simulink library "libbha_parts_bellows"  (R2013b)
settings: Solver=FixedStepDiscrete  StartTime=0.0  StopTime=Inf  FixedStep=0.004  RelTol=1e-3
PostLoadFcn:
  | , if any(exist('dsrtsu_mdlpostloadfcn', 'file') == [2, 3, 6]), try dsrtsu_mdlpostloadfcn('Execute', bdroot); catch fprintf('Error in PostLoadFcn (dsrtsu_mdlpostloadfcn) for model "%s":\n %s\n', bdroot, lasterr); end, end,
undefined symbols (not defined in the file or in its folder): DiscIntNeverNeededParam, p1i
libraries: libbha_parts_bellows x4, libbha_parameters x1
settings Model: DSRTSU_INTERNAL_RTI_VER=440  DSRTSU_INTERNAL_RTI_TYPE=rti1005  DSRTSU_INTERNAL_RTIFPGA=30  Creator=Falkenhahn  LastModifiedBy=fav

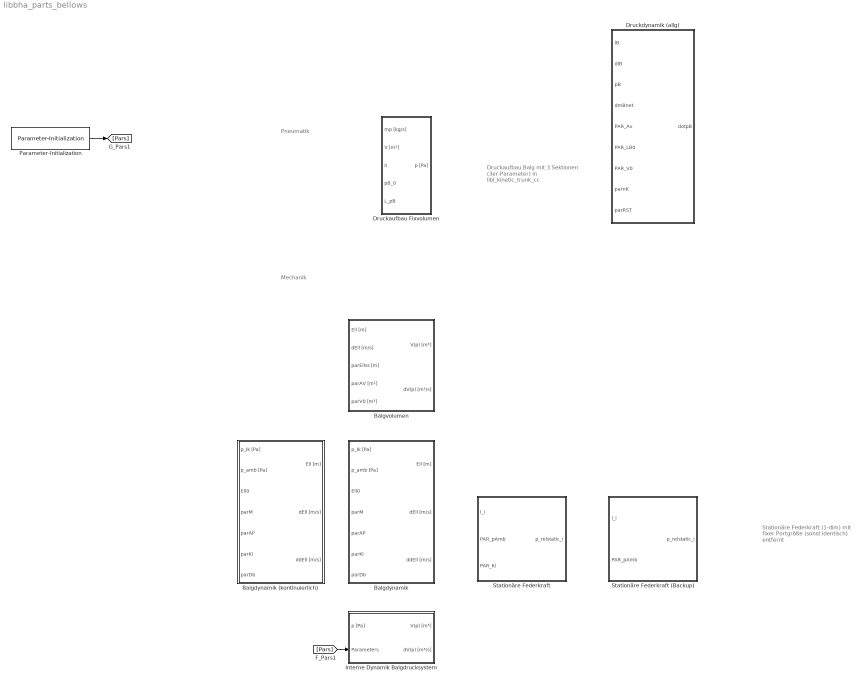
== system libbha_parts_bellows ==
  note: Stationäre Federkraft (1-dim)
      | mit fixer Portgröße (sonst identisch)
      | entfernt
  note: Druckaufbau Balg mit 3 Sektionen
      | (3er-Parameter) in
      | libl_kinetic_trunk_cc
  note: Mechanik
  note: Pneumatik
  Balgdynamik : Subsystem
  Balgdynamik (kontinuierlich) : Subsystem
      settings: AttributesFormatString=|
      | kontinuierliche Integratoren
      | (nicht geeignet für RTW)
  Balgvolumen : Subsystem
  Druckaufbau Fixvolumen : Subsystem  mask{R=288, T0=293.15}
  Druckdynamik (allg) : MATLAB Function  TreatAsAtomicUnit=on
  Interne Dynamik Balgdrucksystem : Subsystem
  Parameter-Initialization : libbha_parameters/Parameter-Initialization  bha_var_choice=BHA  tA=CONST.tA
      settings: AttributesFormatString=|
      | BHA-Variable: %<bha_var_choice>
      | sample time: %<tA>
  Stationäre Federkraft : Subsystem
      settings: AttributesFormatString=|
      | Federkennlinie als Interpolation mittels
      | Polynom 3. Ordnung mit balgspezifischen
      | Parametern p0 (konst) bis p3 (kubisch)
  Stationäre Federkraft (Backup) : Subsystem
      settings: AttributesFormatString=Federkennlinie fest einprogrammiert
  wires:
  Parameter-Initialization/1 -> [Pars]
  [Pars] -> Interne Dynamik Balgdrucksystem/2(Parameters)

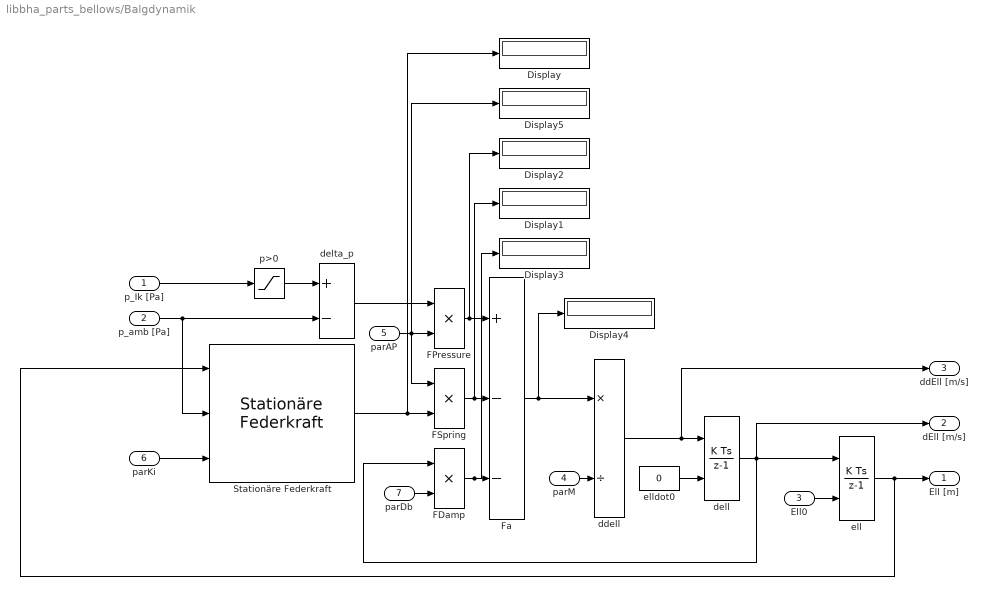
== system libbha_parts_bellows/Balgdynamik ==
  p_Ik [Pa] : Inport
  p_amb [Pa] : Inport  Port=2
  Ell0 : Inport  Port=3
  parM : Inport  Port=4
  parAP : Inport  Port=5
  parKi : Inport  Port=6
      settings: AttributesFormatString=|
      | n x 4
      | n = dim(l)
  parDb : Inport  Port=7
  Display{,1..5} (6 alike) : Display
  FDamp : Product  Inputs=**  OutDataTypeStr=Inherit: Same as first input
  FPressure : Product  Inputs=**  OutDataTypeStr=Inherit: Same as first input
  FSpring : Product  Inputs=**  OutDataTypeStr=Inherit: Same as first input
  Fa : Sum  Inputs=+--  OutDataTypeStr=Inherit: Same as first input
  Stationäre Federkraft : libbha_parts_bellows/Stationäre Federkraft
  ddell : Product  Inputs=*/  OutDataTypeStr=Inherit: Same as first input
  dell : DiscreteIntegrator  InitialConditionSource=external  SampleTime=-1  ICPrevOutput=DiscIntNeverNeededParam  ICPrevScaledInput=DiscIntNeverNeededParam
  delta_p : Sum  Inputs=+-  OutDataTypeStr=Inherit: Same as first input
  ell : DiscreteIntegrator  InitialConditionSource=external  SampleTime=-1  ICPrevOutput=DiscIntNeverNeededParam  ICPrevScaledInput=DiscIntNeverNeededParam
  elldot0 : Constant  Value=0
  p>0 : Saturate  UpperLimit=inf  LowerLimit=0.001e5
  Ell [m] : Outport
  dEll [m/s] : Outport  Port=2
  ddEll [m/s] : Outport  Port=3
  wires:
  Stationäre Federkraft/1 -> Display/1, FSpring/2
  parAP/1 -> FPressure/2, Display5/1, FSpring/1
  parDb/1 -> FDamp/2
  ddell/1 -> dell/1, ddEll [m/s]/1
  parM/1 -> ddell/2
  Fa/1 -> Display4/1, ddell/1
  FPressure/1 -> Display2/1, Fa/1
  p_Ik [Pa]/1 -> p>0/1
  p_amb [Pa]/1 -> Stationäre Federkraft/2, delta_p/2
  delta_p/1 -> FPressure/1
  FSpring/1 -> Fa/2, Display1/1
  FDamp/1 -> Display3/1, Fa/3
  ell/1 -> Ell [m]/1, Stationäre Federkraft/1
  dell/1 -> ell/1, FDamp/1, dEll [m/s]/1
  elldot0/1 -> dell/2
  Ell0/1 -> ell/2
  p>0/1 -> delta_p/1
  parKi/1 -> Stationäre Federkraft/3

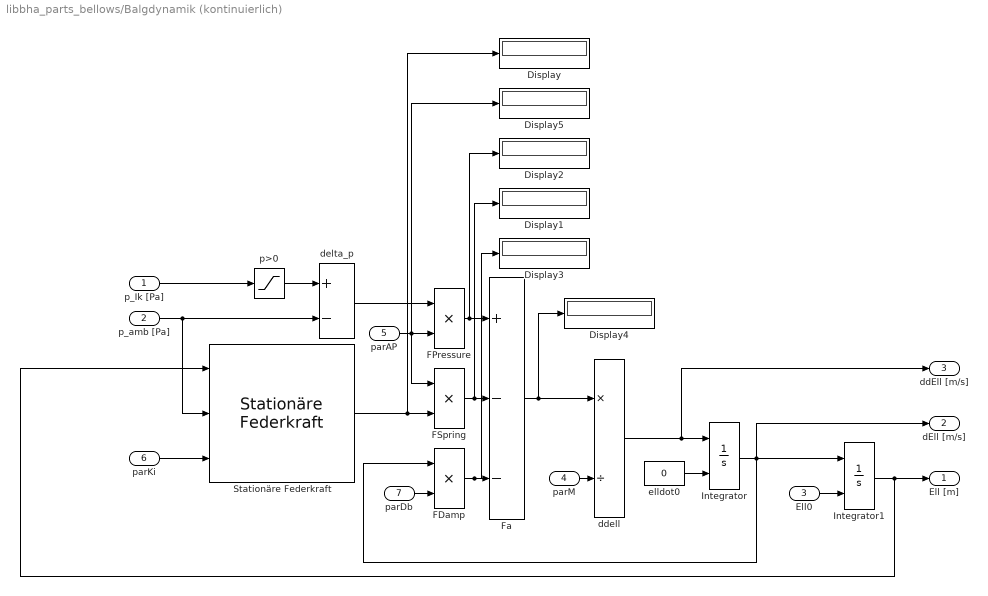
== system libbha_parts_bellows/Balgdynamik (kontinuierlich) ==
  p_Ik [Pa] : Inport
  p_amb [Pa] : Inport  Port=2
  Ell0 : Inport  Port=3
  parM : Inport  Port=4
  parAP : Inport  Port=5
  parKi : Inport  Port=6
      settings: AttributesFormatString=|
      | n x 4
      | n = dim(l)
  parDb : Inport  Port=7
  Display{,1..5} (6 alike) : Display
  FDamp : Product  Inputs=**  OutDataTypeStr=Inherit: Same as first input
  FPressure : Product  Inputs=**  OutDataTypeStr=Inherit: Same as first input
  FSpring : Product  Inputs=**  OutDataTypeStr=Inherit: Same as first input
  Fa : Sum  Inputs=+--  OutDataTypeStr=Inherit: Same as first input
  Integrator : Integrator  InitialConditionSource=external
  Integrator1 : Integrator  InitialConditionSource=external
  Stationäre Federkraft : libbha_parts_bellows/Stationäre Federkraft
  ddell : Product  Inputs=*/  OutDataTypeStr=Inherit: Same as first input
  delta_p : Sum  Inputs=+-  OutDataTypeStr=Inherit: Same as first input
  elldot0 : Constant  Value=0
  p>0 : Saturate  UpperLimit=inf  LowerLimit=0.001e5
  Ell [m] : Outport
  dEll [m/s] : Outport  Port=2
  ddEll [m/s] : Outport  Port=3
  wires:
  parKi/1 -> Stationäre Federkraft/3
  p>0/1 -> delta_p/1
  Ell0/1 -> Integrator1/2
  elldot0/1 -> Integrator/2
  Integrator/1 -> Integrator1/1, dEll [m/s]/1, FDamp/1
  Integrator1/1 -> Stationäre Federkraft/1, Ell [m]/1
  FDamp/1 -> Fa/3, Display3/1
  FSpring/1 -> Display1/1, Fa/2
  delta_p/1 -> FPressure/1
  p_amb [Pa]/1 -> delta_p/2, Stationäre Federkraft/2
  p_Ik [Pa]/1 -> p>0/1
  FPressure/1 -> Fa/1, Display2/1
  Fa/1 -> ddell/1, Display4/1
  parM/1 -> ddell/2
  ddell/1 -> Integrator/1, ddEll [m/s]/1
  parDb/1 -> FDamp/2
  parAP/1 -> FSpring/1, Display5/1, FPressure/2
  Stationäre Federkraft/1 -> FSpring/2, Display/1

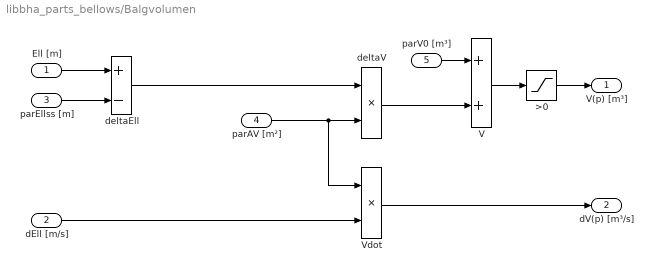
== system libbha_parts_bellows/Balgvolumen ==
  Ell [m] : Inport
  dEll [m/s] : Inport  Port=2
  parEllss [m] : Inport  Port=3
  parAV [m²] : Inport  Port=4
  parV0 [m³] : Inport  Port=5
  >0 : Saturate  UpperLimit=inf  LowerLimit=0.1e-6
  V : Sum
  Vdot : Product  Inputs=**
  deltaEll : Sum  Inputs=+-
  deltaV : Product  Inputs=**
  V(p) [m³] : Outport
  dV(p) [m³/s] : Outport  Port=2
  wires:
  deltaV/1 -> V/2
  parEllss [m]/1 -> deltaEll/2
  Ell [m]/1 -> deltaEll/1
  >0/1 -> V(p) [m³]/1
  parAV [m²]/1 -> deltaV/2, Vdot/1
  Vdot/1 -> dV(p) [m³/s]/1
  V/1 -> >0/1
  parV0 [m³]/1 -> V/1
  deltaEll/1 -> deltaV/1
  dEll [m/s]/1 -> Vdot/2

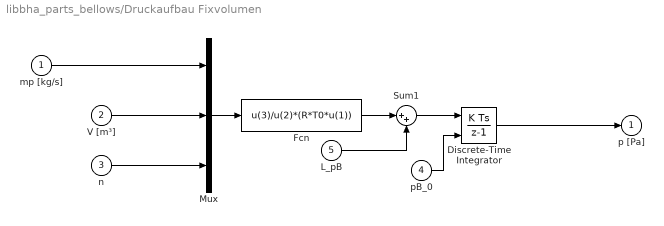
== system libbha_parts_bellows/Druckaufbau Fixvolumen ==
  mp [kg/s] : Inport
  V [m³] : Inport  Port=2
  n : Inport  Port=3
  pB_0 : Inport  Port=4
  L_pB : Inport  Port=5
  Discrete-Time Integrator : DiscreteIntegrator  InitialConditionSource=external  InitialCondition=p1i  SampleTime=-1  ICPrevOutput=DiscIntNeverNeededParam  ICPrevScaledInput=DiscIntNeverNeededParam
  Fcn : Fcn  Expr=u(3)/u(2)*(R*T0*u(1))
  Mux : Mux  Inputs=3
  Sum1 : Sum  Inputs=|++
  p [Pa] : Outport  InitialOutput=0
  wires:
  L_pB/1 -> Sum1/2
  pB_0/1 -> Discrete-Time Integrator/2
  Sum1/1 -> Discrete-Time Integrator/1
  Discrete-Time Integrator/1 -> p [Pa]/1
  Mux/1 -> Fcn/1
  mp [kg/s]/1 -> Mux/1
  Fcn/1 -> Sum1/1
  V [m³]/1 -> Mux/2
  n/1 -> Mux/3

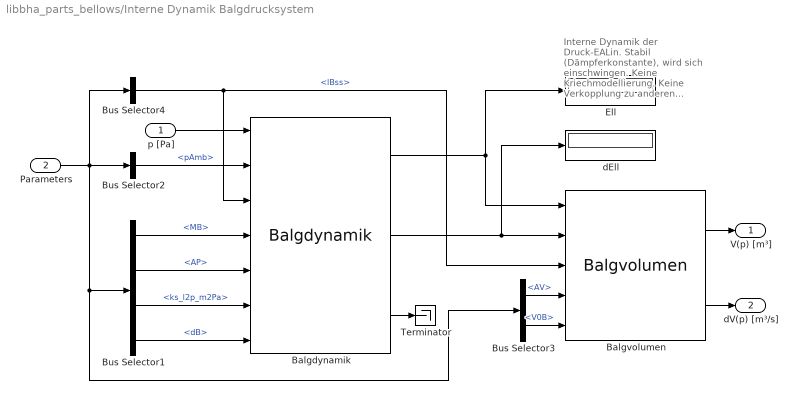
== system libbha_parts_bellows/Interne Dynamik Balgdrucksystem ==
  note: Interne Dynamik der Druck-EALin.
      | Stabil (Dämpferkonstante), wird sich einschwingen.
      | Keine Kriechmodellierung. Keine Verkopplung zu anderen Bälgen.
  p [Pa] : Inport
  Parameters : Inport  Port=2
  Balgdynamik : libbha_parts_bellows/Balgdynamik
  Balgvolumen : libbha_parts_bellows/Balgvolumen
  Bus Selector1 : BusSelector  OutputSignals=Bellows.MB,Bellows.AP,Bellows.ks_l2p_m2Pa,Bellows.dB
  Bus Selector2 : BusSelector  OutputSignals=Pressure.pAmb
  Bus Selector3 : BusSelector  OutputSignals=Bellows.AV,Bellows.V0B
  Bus Selector4 : BusSelector  OutputSignals=Bellows.lBss
  Ell : Display
  Terminator : Terminator
  dEll : Display
  V(p) [m³] : Outport
  dV(p) [m³/s] : Outport  Port=2
  wires:
  Bus Selector2/1 -> Balgdynamik/2  "<pAmb>"
  p [Pa]/1 -> Balgdynamik/1
  Balgvolumen/2 -> dV(p) [m³/s]/1
  Balgvolumen/1 -> V(p) [m³]/1
  Balgdynamik/1 -> Ell/1, Balgvolumen/1
  Balgdynamik/2 -> dEll/1, Balgvolumen/2
  Balgdynamik/3 -> Terminator/1
  Bus Selector4/1 -> Balgdynamik/3, Balgvolumen/3  "<lBss>"
  Parameters/1 -> Bus Selector3/1, Bus Selector1/1, Bus Selector4/1, Bus Selector2/1
  Bus Selector1/2 -> Balgdynamik/5  "<AP>"
  Bus Selector1/1 -> Balgdynamik/4  "<MB>"
  Bus Selector1/4 -> Balgdynamik/7  "<dB>"
  Bus Selector3/1 -> Balgvolumen/4  "<AV>"
  Bus Selector3/2 -> Balgvolumen/5  "<V0B>"
  Bus Selector1/3 -> Balgdynamik/6  "<ks_l2p_m2Pa>"

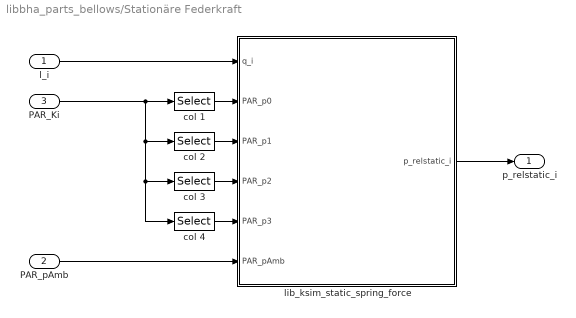
== system libbha_parts_bellows/Stationäre Federkraft ==
  l_i : Inport
  PAR_pAmb : Inport  Port=2
  PAR_Ki : Inport  Port=3
      settings: AttributesFormatString=|
      | Parametermatrix mit Koeffizienten
      | für Federkraftinterpolation
      | 
      | 4 Spalten mit p0 p1 p2 p3
      | n Zeilen (für jeden Balg)
  col 1 : Selector  NumberOfDimensions=2  InputPortWidth=3  IndexOptions=Select all,Index vector (dialog)  Indices=[1 3],1  OutputSizes=1,1
  col 2 : Selector  NumberOfDimensions=2  InputPortWidth=3  IndexOptions=Select all,Index vector (dialog)  Indices=[1 3],2  OutputSizes=1,1
  col 3 : Selector  NumberOfDimensions=2  InputPortWidth=3  IndexOptions=Select all,Index vector (dialog)  Indices=[1 3],3  OutputSizes=1,1
  col 4 : Selector  NumberOfDimensions=2  InputPortWidth=3  IndexOptions=Select all,Index vector (dialog)  Indices=[1 3],4  OutputSizes=1,1
  lib_ksim_static_spring_force : MATLAB Function  TreatAsAtomicUnit=on
  p_relstatic_i : Outport
  wires:
  lib_ksim_static_spring_force/1(p_relstatic_i) -> p_relstatic_i/1
  PAR_pAmb/1 -> lib_ksim_static_spring_force/6(PAR_pAmb)
  l_i/1 -> lib_ksim_static_spring_force/1(q_i)
  col 1/1 -> lib_ksim_static_spring_force/2(PAR_p0)
  col 3/1 -> lib_ksim_static_spring_force/4(PAR_p2)
  col 4/1 -> lib_ksim_static_spring_force/5(PAR_p3)
  col 2/1 -> lib_ksim_static_spring_force/3(PAR_p1)
  PAR_Ki/1 -> col 2/1, col 3/1, col 4/1, col 1/1

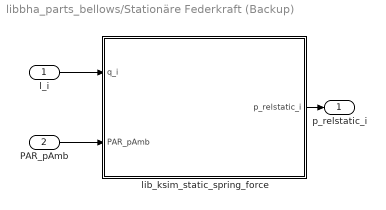
== system libbha_parts_bellows/Stationäre Federkraft (Backup) ==
  l_i : Inport
  PAR_pAmb : Inport  Port=2
  lib_ksim_static_spring_force : MATLAB Function  TreatAsAtomicUnit=on
  p_relstatic_i : Outport
  wires:
  l_i/1 -> lib_ksim_static_spring_force/1(q_i)
  PAR_pAmb/1 -> lib_ksim_static_spring_force/2(PAR_pAmb)
  lib_ksim_static_spring_force/1(p_relstatic_i) -> p_relstatic_i/1

== matlab function libbha_parts_bellows/Stationäre Federkraft (Backup)/lib_ksim_static_spring_force ==
  data: p_relstatic_i output; q_i input; PAR_pAmb input size=1
function p_relstatic_i   = kff_forces(q_i, PAR_pAmb)

%function p_relstatic_i   = kff_forces(q_i, ~, ~, PAR_pAmb)
%%%
%%%   ACHTUNG: stationäre Federkraft/ stationärer Druck nie mit Steifigkeitskennlinie und Parameter BHA.Kin.l_ik_init initialisieren
%%%            Kriechverhalten darf nicht die Initialisierungslänge (Volumenänderung!) verändern.
%%%


%
% Parameter
%   - mode              [unused] Schalter zum Definieren der Modi
%   - PAR_SecNum        [unused] Sektionsnummer
%   - PAR_pAmb                   Umgebungsdruck

    %#codegen

    
    %% Federkraft aus Lookuptabelle mit linearer Extrapolation
    % Stand 2013-11
    % Absoluter Druck über absoluter Länge
    
%     % Nur quasilinearer Teil der Kennlinie ohne "auf-Block-fahren"
%     %PAR_lt_l = [0.1707;0.1755;0.1802;0.1853;0.1906;0.1961;0.2015;0.2068;0.2122;0.2175;0.2227;0.2277;0.2324;0.2371;0.2417;0.2461;0.2502;0.2544;0.2583;0.2621;0.2658;0.2695;0.2728;0.2767;0.2803];
%     %PAR_lt_p = [85064;90057;95042;100042;105031;110032;115029;120023;125016;130011;135005;140000;144995;149987;154982;159976;164974;169967;174962;179959;184959;189947;194941;199833;204790];
%     
%     % Steil abflachende, aufgenommene Kurve. Bei Unterdruck keine
%     % Längenänderung mehr vorhanden
%     PAR_lt_l = [0.16768;0.16774;0.16798;0.16811;0.16828;0.16884;0.16982;0.1707;0.1755;0.1802;0.1853;0.1906;0.1961;0.2015;0.2068;0.2122;0.2175;0.2227;0.2277;0.2324;0.2371;0.2417;0.2461;0.2502;0.2544;0.2583;0.2621;0.2658;0.2695;0.2728;0.2767;0.2803];
%     PAR_lt_p = [55080;70074;75061;79990;81483;82985;84485;85064;90057;95042;100042;105031;110032;115029;120023;125016;130011;135005;140000;144995;149987;154982;159976;164974;169967;174962;179959;184959;189947;194941;199833;204790];
%     
%     if q_i < PAR_lt_l(1) % Lineare Extrapolation für kleinere Werte
%         p_relstatic_i = (PAR_lt_p(2) - PAR_lt_p(1))/(PAR_lt_l(2) - PAR_lt_l(1)) * (q_i - PAR_lt_l(1)) + PAR_lt_p(1) - PAR_pAmb; 
%     elseif q_i > PAR_lt_l(end) % Lineare Extrapolation für größere Werte
%         p_relstatic_i = (PAR_lt_p(end) - PAR_lt_p(end-1))/(PAR_lt_l(end) - PAR_lt_l(end-1)) * (q_i - PAR_lt_l(end-1)) + PAR_lt_p(end-1) - PAR_pAmb;
%     else
%         p_relstatic_i = interp1(PAR_lt_l, PAR_lt_p, q_i, 'linear') - PAR_pAmb;
%     end
    
    %% Federkraft aus Fitfunktion (v0) [Mahl]
    % Stand 2012-12
      
%     PAR_c_Balg_lin = 1e3*[ 944.0; 831.7; 892.1];
%     PAR_c_Balg_sqr = 1e4*[ 392.4; 357.5; 233.3];
%     delta_l = (q_i - 0.174);
%     p_relstatic_i   = delta_l .* PAR_c_Balg_lin(PAR_SecNum) + delta_l.^2 .* PAR_c_Balg_sqr(PAR_SecNum);

    %% Federkraft aus Fitfunktion (v1)
    % Stand 2013-01
    
%     PAR_c_FFB5 = [ 7.453e5 -4.758e4 1.133e8 -1.797e9 9.122e9 ];
%     delta_l = (q_i - 0.174);
%     p_relstatic_i = PAR_c_FFB5(1)*delta_l + PAR_c_FFB5(2)*delta_l^2 + PAR_c_FFB5(3)*delta_l^3 + PAR_c_FFB5(4)*delta_l^4 + PAR_c_FFB5(5)*delta_l^5;
    
    %% Federkraft aus Fitfunktion (v2)
    % Stand 2013-11
    % Absoluter Druck über absoluter Länge
    
    PAR_c_FFB5 = [ -1.987e+06; 3.8e+07; -2.783e+08; 1.009e+09; -1.763e+09; 1.197e+09 ];
    p_relstatic_i = PAR_c_FFB5(1) + PAR_c_FFB5(2)*q_i + PAR_c_FFB5(3)*q_i.^2 + PAR_c_FFB5(4)*q_i.^3 + PAR_c_FFB5(5)*q_i.^4 + PAR_c_FFB5(6)*q_i.^5 - PAR_pAmb;
    

end

== matlab function libbha_parts_bellows/Druckdynamik (allg) ==
  data: lB input; dotpB output; dlB input; pB input; dmBnet input; PAR_Av input; PAR_LB0 input; PAR_V0 input; parnK input size=1; parRST input size=1
function dotpB = ksim_pressure(lB, dlB, pB, dmBnet, PAR_Av, PAR_LB0, PAR_V0, parnK, parRST)

    dotpB = parnK./(PAR_Av.*(lB-PAR_LB0)+PAR_V0) .* (parRST*dmBnet - PAR_Av.*dlB.*pB);

end

== matlab function libbha_parts_bellows/Stationäre Federkraft/lib_ksim_static_spring_force ==
  data: p_relstatic_i output; q_i input; PAR_p0 input; PAR_p1 input; PAR_p2 input; PAR_p3 input; PAR_pAmb input size=1
function p_relstatic_i   = kff_forces(q_i, PAR_p0, PAR_p1, PAR_p2, PAR_p3, PAR_pAmb)
%%%   ACHTUNG: stationäre Federkraft/ stationärer Druck nie mit Steifigkeitskennlinie und Parameter BHA.Kin.l_ik_init initialisieren
%%%            Kriechverhalten darf nicht die Initialisierungslänge (Volumenänderung!) verändern.

    %p_relstatic_i =  PAR_p0.*ones(9,1) + PAR_p1.*q_i + PAR_p2.*q_i.^2  + PAR_p3.*q_i.^3 - PAR_pAmb;
    % if numel(PAR_p0) == 1 && numel(q_i) > 1 -> als skalare verwenden
    p_relstatic_i =  PAR_p0 + PAR_p1.*q_i + PAR_p2.*q_i.^2  + PAR_p3.*q_i.^3 - PAR_pAmb;

end


%% Alte Versionen als Kommentare unten im Quelltext
    
    %% Federkraft aus Lookuptabelle mit linearer Extrapolation
    % Stand 2013-11
    % Absoluter Druck über absoluter Länge
    
%     % Nur quasilinearer Teil der Kennlinie ohne "auf-Block-fahren"
%     %PAR_lt_l = [0.1707;0.1755;0.1802;0.1853;0.1906;0.1961;0.2015;0.2068;0.2122;0.2175;0.2227;0.2277;0.2324;0.2371;0.2417;0.2461;0.2502;0.2544;0.2583;0.2621;0.2658;0.2695;0.2728;0.2767;0.2803];
%     %PAR_lt_p = [85064;90057;95042;100042;105031;110032;115029;120023;125016;130011;135005;140000;144995;149987;154982;159976;164974;169967;174962;179959;184959;189947;194941;199833;204790];
%     
%     % Steil abflachende, aufgenommene Kurve. Bei Unterdruck keine
%     % Längenänderung mehr vorhanden
%     PAR_lt_l = [0.16768;0.16774;0.16798;0.16811;0.16828;0.16884;0.16982;0.1707;0.1755;0.1802;0.1853;0.1906;0.1961;0.2015;0.2068;0.2122;0.2175;0.2227;0.2277;0.2324;0.2371;0.2417;0.2461;0.2502;0.2544;0.2583;0.2621;0.2658;0.2695;0.2728;0.2767;0.2803];
%     PAR_lt_p = [55080;70074;75061;79990;81483;82985;84485;85064;90057;95042;100042;105031;110032;115029;120023;125016;130011;135005;140000;144995;149987;154982;159976;164974;169967;174962;179959;184959;189947;194941;199833;204790];
%     
%     if q_i < PAR_lt_l(1) % Lineare Extrapolation für kleinere Werte
%         p_relstatic_i = (PAR_lt_p(2) - PAR_lt_p(1))/(PAR_lt_l(2) - PAR_lt_l(1)) * (q_i - PAR_lt_l(1)) + PAR_lt_p(1) - PAR_pAmb; 
%     elseif q_i > PAR_lt_l(end) % Lineare Extrapolation für größere Werte
%         p_relstatic_i = (PAR_lt_p(end) - PAR_lt_p(end-1))/(PAR_lt_l(end) - PAR_lt_l(end-1)) * (q_i - PAR_lt_l(end-1)) + PAR_lt_p(end-1) - PAR_pAmb;
%     else
%         p_relstatic_i = interp1(PAR_lt_l, PAR_lt_p, q_i, 'linear') - PAR_pAmb;
%     end
    
    %% Federkraft aus Fitfunktion (v0) [Mahl]
    % Stand 2012-12
      
%     PAR_c_Balg_lin = 1e3*[ 944.0; 831.7; 892.1];
%     PAR_c_Balg_sqr = 1e4*[ 392.4; 357.5; 233.3];
%     delta_l = (q_i - 0.174);
%     p_relstatic_i   = delta_l .* PAR_c_Balg_lin(PAR_SecNum) + delta_l.^2 .* PAR_c_Balg_sqr(PAR_SecNum);

    %% Federkraft aus Fitfunktion (v1)
    % Stand 2013-01
    
%     PAR_c_FFB5 = [ 7.453e5 -4.758e4 1.133e8 -1.797e9 9.122e9 ];
%     delta_l = (q_i - 0.174);
%     p_relstatic_i = PAR_c_FFB5(1)*delta_l + PAR_c_FFB5(2)*delta_l^2 + PAR_c_FFB5(3)*delta_l^3 + PAR_c_FFB5(4)*delta_l^4 + PAR_c_FFB5(5)*delta_l^5;
    
    %% Federkraft aus Fitfunktion (v2)
    % Stand 2013-11
    % Absoluter Druck über absoluter Länge
    
%    PAR_c_FFB5 = [ -1.987e+06; 3.8e+07; -2.783e+08; 1.009e+09; -1.763e+09; 1.197e+09 ];
%    p_relstatic_i = PAR_c_FFB5(1) + PAR_c_FFB5(2)*q_i + PAR_c_FFB5(3)*q_i.^2 + PAR_c_FFB5(4)*q_i.^3 + PAR_c_FFB5(5)*q_i.^4 + PAR_c_FFB5(6)*q_i.^5 - PAR_pAmb;
